simulink model "untitled"  (R2025a)
settings: Solver=VariableStepAuto  StartTime=0.0  StopTime=10.0  RelTol=1e-3
values from neighbouring files (symbols this model uses):
  alfa = cos(0.34906585)    [parameters.m]
  B_m = 0.000001    (= 1e-06)    [parameters.m]
  compare_to_volt = 0.01171875    [parameters.m]
  g = 9.8    [parameters.m]
  Gr = 1/30    (= 0.0333333333333)    [parameters.m]
  J_m = 0.000004    (= 4e-06)    [parameters.m]
  K_t = 0.01    [parameters.m]
  L_a = 0.0048436939    [parameters.m]
  m = 0.1    [parameters.m]
  R = 0.017    [parameters.m]
  R_a = 2.2    [parameters.m]
  tick_p_meter = 17975.15    [parameters.m]
libraries: slpidlib x1
settings Model: Creator=55419  LastModifiedBy=bruno

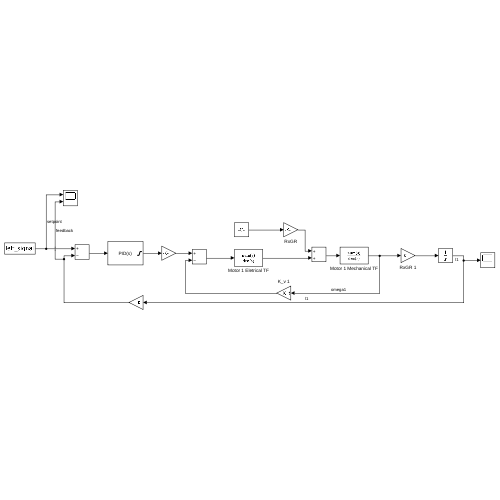
[thumbnail: Simulink's stored preview of the top-level diagram]
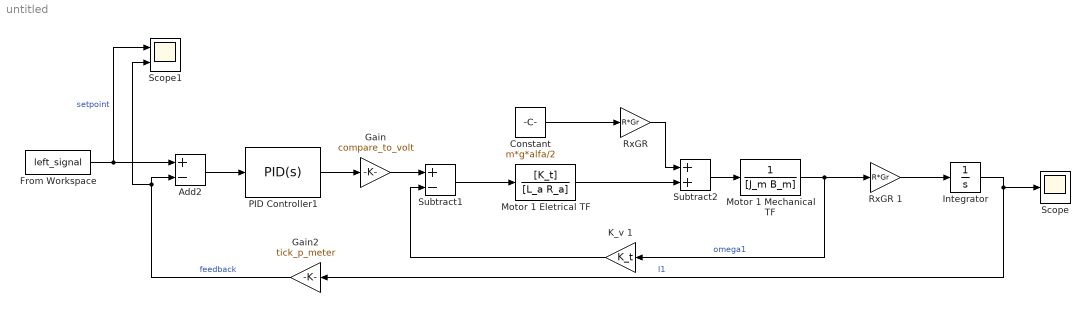
== system untitled ==
  Add2 : Sum  Inputs=+-
  Constant : Constant  Value=m*g*alfa/2
  From Workspace : FromWorkspace  VariableName=left_signal  OutputAfterFinalValue=Holding final value
  Gain : Gain  Gain=compare_to_volt
  Gain2 : Gain  Gain=tick_p_meter
  Integrator : Integrator  InitialCondition=0.4272
  K_v 1 : Gain  Gain=K_t
  Motor 1 Eletrical TF : TransferFcn  Numerator=[K_t]  Denominator=[L_a R_a]
  Motor 1 Mechanical TF : TransferFcn  Denominator=[J_m B_m]
  PID Controller1 : slpidlib/PID Controller  Controller=PID  Form=Parallel  TimeDomain=Continuous-time  UseExternalTs=off  SampleTime=-1  IntegratorMethod=Forward Euler  FilterMethod=Forward Euler  ControllerParametersSource=internal  P=12.4904214867502  I=55.0268356378833  UseKiTs=off  D=0.706999336768987  UseExternalDerivativeSource=off  N=11016.6397995038  UseFilter=on  TunerSelectOption=Transfer Function Based (PID Tuner App)  InitialConditionSource=internal  InitialConditionForIntegrator=0  InitialConditionForFilter=0  DifferentiatorICPrevScaledInput=0  ExternalReset=none  TrackingMode=off  Kt=1  LimitOutput=on  SatLimitsSource=internal  UpperSaturationLimit=1024  LowerSaturationLimit=-1024  LinearizeAsGain=off  AntiWindupMode=none  Kb=1  LimitIntegrator=off  UpperIntegratorSaturationLimit=inf  LowerIntegratorSaturationLimit=-inf  POutMin=[]  POutMax=[]  IOutMin=[]  IOutMax=[]  DOutMin=[]  DOutMax=[]  NOutMin=[]  NOutMax=[]  SumOutMin=[]  SumOutMax=[]  SaturationOutMin=[]  SaturationOutMax=[]  PParamMin=[]  PParamMax=[]  IParamMin=[]  IParamMax=[]  DParamMin=[]  DParamMax=[]  NParamMin=[]  NParamMax=[]  KbParamMin=[]  KbParamMax=[]  KtParamMin=[]  KtParamMax=[]  KbOutMin=[]  KbOutMax=[]  KtOutMin=[]  KtOutMax=[]  IntegratorOutMin=[]  IntegratorOutMax=[]  FilterOutMin=[]  FilterOutMax=[]  SumI1OutMin=[]  SumI1OutMax=[]  SumI2OutMin=[]  SumI2OutMax=[]  SumI3OutMin=[]  SumI3OutMax=[]  SumI4OutMin=[]  SumI4OutMax=[]  SumDOutMin=[]  SumDOutMax=[]  DifferentiatorOutMin=[]  DifferentiatorOutMax=[]  FilterDiffOutCoefMin=[]  FilterDiffOutCoefMax=[]  ReciprocalOutMin=[]  ReciprocalOutMax=[]  SumDenOutMin=[]  SumDenOutMax=[]  SumNumOutMin=[]  SumNumOutMax=[]  DivideOutMin=[]  DivideOutMax=[]  UdiffTsProdOutMin=[]  UdiffTsProdOutMax=[]  NTsProdOutMin=[]  NTsProdOutMax=[]  UintegralTsProdOutMin=[]  UintegralTsProdOutMax=[]  UngainTsProdOutMin=[]  UngainTsProdOutMax=[]  ClampingZeroOutDataTypeStr=Inherit: Inherit via back propagation  ClampingZeroOutMin=[]  ClampingZeroOutMax=[]  FilterDenConstantOutDataTypeStr=Inherit: Inherit via back propagation  FilterDenConstantOutMin=[]  FilterDenConstantOutMax=[]  PCopyOutDataTypeStr=Inherit: Inherit via back propagation  PCopyOutMin=[]  PCopyOutMax=[]  NCopyOutDataTypeStr=Inherit: Inherit via back propagation  NCopyOutMin=[]  NCopyOutMax=[]  IntegratorContinuousStateAttributes=''  IntegratorStateMustResolveToSignalObject=off  IntegratorRTWStateStorageClass=Auto  FilterContinuousStateAttributes=''  FilterStateMustResolveToSignalObject=off  FilterRTWStateStorageClass=Auto  ParallelPVariant=InternalParameters  IdealPVariant=Disabled  IVariant=InternalParameters  DVariant=InternalParameters  IntegratorVariant=Continuous  SatVariant=Enabled  AWVariant=Passthrough  PCopyVariant=Disabled  TRVariant=Disabled  FdbkBlocksVariant=Forward  IdealPFdbkVariant=Disabled  SatFdbkVariant=Disabled  DerivativeFilterVariant=ContFilter  NVariant=InternalParameters  NCopyVariant=Disabled  FilterICVariant=InternalICsFilter  IntegratorICVariant=InternalICs  ExternalResetVariant=Disabled  TRSumVariant=Passthrough  SumFdbkVariant=Disabled  SumVariant=Sum_PID  TsampFilterVariant=InternalTs  TsampNgainVariant=Passthrough  TsampIntegralVariant=Disabled_SignalSpec  ExternalSaturationOutDataTypeStr=Inherit: Same as second input  DerivativeSourceVariant=ErrorSignal  PreIntVariant=InternalPreInt
  RxGR : Gain  Gain=R*Gr
  RxGR 1 : Gain  Gain=R*Gr
  Scope : Scope
      settings: ActiveDisplayYMinimum=0.22945866819317454  ActiveDisplayYMaximum=0.76743839294883276
  Scope1 : Scope  NumInputPorts=2
      settings: ActiveDisplayYMinimum=-5637.0079598408774  ActiveDisplayYMaximum=75781.122082504851
  Subtract1 : Sum  Inputs=+-
  Subtract2 : Sum
  wires:
  Gain2/1 -> Scope1/2, Add2/2  "feedback"
  K_v 1/1 -> Subtract1/2
  Subtract1/1 -> Motor 1 Eletrical TF/1
  RxGR/1 -> Subtract2/1
  Motor 1 Mechanical TF/1 -> RxGR 1/1, K_v 1/1  "omega1"
  Subtract2/1 -> Motor 1 Mechanical TF/1
  Motor 1 Eletrical TF/1 -> Subtract2/2
  RxGR 1/1 -> Integrator/1
  Add2/1 -> PID Controller1/1
  From Workspace/1 -> Scope1/1, Add2/1  "setpoint"
  Integrator/1 -> Scope/1, Gain2/1  "l1"
  PID Controller1/1 -> Gain/1
  Constant/1 -> RxGR/1
  Gain/1 -> Subtract1/1
